simulink model "symulink_identool_error_model"  (Simulink 7.7)
settings: Solver=ode45  StartTime=0.0  StopTime=ttfin  RelTol=1e-3
values from neighbouring files (symbols this model uses):
  Ko = (Yf-Yo)/(Uf-Uo)    [IDFOM.m]
  kpp = koo/0.001    [IDFOM.m]
  Lo = xns(3)    [IDFOM.m]
  tmax = max(tnorm)    [IDFOM.m]
  tuin = Yo/Ko    [IDFOM.m]
  Uf = mean(u(long-sample+1:long))    [IDFOM.m]
  Uo = mean(u(1:sample))    [IDFOM.m]
undefined symbols (not defined in the file or in its folder): po, zo
settings Model: Creator=Eguevara  LastModifiedBy=helber
settings SolverCC: MaxConsecutiveMinStep=ttfin*4

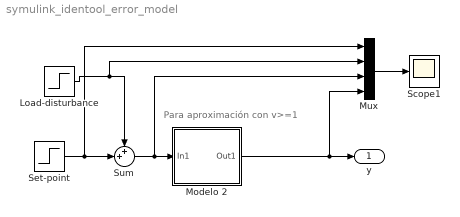
== system symulink_identool_error_model ==
  note: Para aproximación con v>=1
  Load-disturbance : Step  Time=tmax  After=(Uf-Uo)  SampleTime=0.25
  Modelo 2 : Subsystem  mask("FOMPDT" Modelo de orden fraccional más tiempo muerto.       ){z=[zo(1) zo(2) zo(3) zo(4) zo(5) zo(6) zo(7) zo(8) zo(9)], P=[po(1) po(2) po(3) po(4) po(5) po(6) po(7) po(8) po(9)], kpp=kpp, Ko=Ko, Lo=Lo}
      mask prompts: z "Zeros:"; P "Poles:"; kpp "Ganancia de la aproximación "ko":"; Ko "Ganancia del modelo "Ko":"; Lo "Tiempo muerto del modelo "Lo":"
      mask help: Introduzca el valor de los parámetros del modelo de la forma Gm(s)=K*exp(-Ls)/(Ts^v+1). Donde "Ts^v" corresponde a los polos y ceros de la aproximación de cronPadula2modied.
      mask Display: disp('FOMPDT')
  Mux : Mux
  Scope1 : Scope
      settings: TimeRange=3000  YMin=0  YMax=80  SaveName=sc3  DataFormat=Array  MaxDataPoints=1000000
  Set-point : Step  Time=0  After=tuin  SampleTime=0.25
  Sum : Sum  Inputs=++|
  y : Outport
  wires:
  Sum/1 -> Modelo 2/1(In1), Mux/3
  Modelo 2/1(Out1) -> y/1, Mux/4
  Set-point/1 -> Sum/2, Mux/1
  Mux/1 -> Scope1/1
  Load-disturbance/1 -> Sum/1, Mux/2

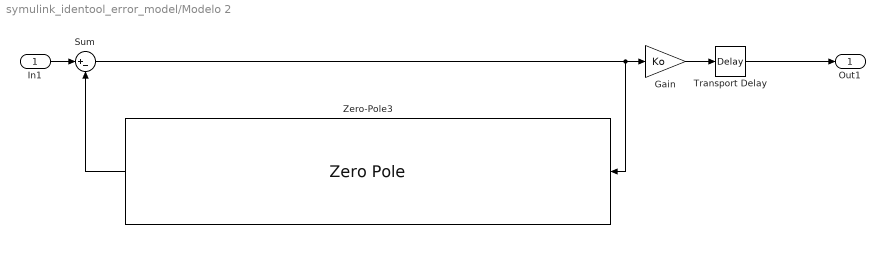
== system symulink_identool_error_model/Modelo 2 ==
  In1 : Inport
  Gain : Gain  Gain=Ko
  Sum : Sum  Inputs=|+-
  Transport Delay : TransportDelay  DelayTime=Lo
  Zero-Pole3 : ZeroPole  Zeros=[zo(1) zo(2) zo(3) zo(4) zo(5) zo(6) zo(7) zo(8) zo(9)]  Poles=[po(1) po(2) po(3) po(4) po(5) po(6) po(7) po(8) po(9)]  Gain=kpp
  Out1 : Outport
  wires:
  Zero-Pole3/1 -> Sum/2
  Sum/1 -> Zero-Pole3/1, Gain/1
  In1/1 -> Sum/1
  Gain/1 -> Transport Delay/1
  Transport Delay/1 -> Out1/1
